simulink library "lpvlibrary"  (R2018b)
settings: Solver=ode45  StartTime=0.0  StopTime=10.0  RelTol=1e-3  EnableMultiTasking=on
values from neighbouring files (symbols this model uses):
  ns = order(pdG)    [lpvctrl.m]    (also in lpvctrl_2.m = size(akh,1); pcss_Sfunction.m = order(sys))
  nu = length(pdG.InputGroup.ctrl)    [lpvctrl.m]    (also in lpvctrl_2.m; test_lpvanalysis.m = 0:10)
  ny = 0    [lft_pass.m]    (also in lft_pgss.m; lft_ppss.m; lpvctrl.m = length(pdG.OutputGroup.meas); lpvctrl_2.m = length(pdG.OutputGroup.meas))
  pdG = pgss(Ap,Bp,C1,0,pv,fcn,'InputName','u','OutputName','y')    [TwoLink_nl.m]    (also in test_lpvanalysis.m = pgss(Acl,B,C,D,pv,func,     'InputName','u',     'OutputName)
undefined symbols (not defined in the file or in its folder): pass, pcss
libraries: $bdroot x10
Description:
  | LPV model library
settings Model: Creator=Fernando  LastModifiedBy=ferna
settings DataIOCC: LimitDataPoints=on
settings OptimizationCC: LifeSpan=inf
settings DebuggingCC: AllowSymbolicDim=off  SFUnexpectedBacktrackingDiag=warning  SFNoUnconditionalDefaultTransitionDiag=warning
settings SFSimCC: SimUseLocalCustomCode=off
settings RTWCC: RTWUseLocalCustomCode=off
settings CodeAppCC: StateflowObjectComments=on
settings GRTTargetCC: TargetLangStandard=C89/C90 (ANSI)  GeneratePreprocessorConditionals=Disable all
settings ConfigComp: CovMetricSettings=dw  CovHtmlReporting=on  CovSaveCumulativeToWorkspaceVar=on  CovSaveSingleToWorkspaceVar=on  CovExternalEMLEnable=off

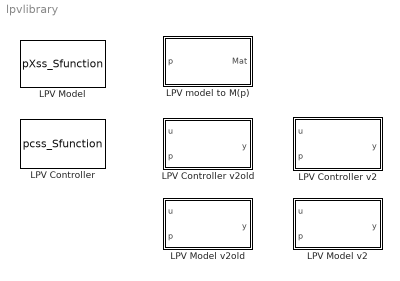
== system lpvlibrary ==
  LPV Controller : M-S-Function  FunctionName=pcss_Sfunction  Parameters=pdSys, x0  mask{pdSys=pcss('demo'), x0=0}
      mask prompts: pdSys "LPV controller (ctrlss)"; x0 "Initial Conditions"
      mask Display:
      | disp('')
      | port_label('input', 1, 'u')
      | port_label('input', 2, 'p')
      | port_label('output', 1, 'y')
  LPV Controller v2 : Subsystem  mask(LPV controller){pdK=pcss('demo'), x0=0}
      mask prompts: pdK "LPV Controller"; x0 "Initial conditions"
      mask help:
      | Online implementation of LPV controller for parameter dependent Lyapunov functions given in an object pcss.
      | Faster implementation than LPV controller block
      mask init:
      | % model dimensions
      | [ny,nu,ns] = size(pdK);
      | 
      | % Lyapunov function at par
      | flagX = isnumeric(pdK.xFcn);
      | flagY = isnumeric(pdK.yFcn);
      | 
      | % DirectFeedthrough flag
      | fDF = any(pdK.ctrller.D(:));
      | if fDF
      |     p1 = find_system(gcb);
      |     p2 = [p1{1} '/Du'];
      |     h1 = get_param(p2,'LineHandles');
      |     delete_line(h1.Outport);
      |     
      |     p1 = find_system(gcb);
      |     p2 = [p1{1} '/d0'];
      |     h1 = get_param(p2,'LineHandles');
      |     delete_line(h1.Outport)
      |     
      |     add_line(gcb,'Du/1','sb/2','autorouting','on');
      |     add_line(gcb,'d0/1','end/1','autorouting','on');
      |        
      | else
      |     p1 = find_system(gcb);
      |     p2 = [p1{1} '/Du'];
      |     h1 = get_param(p2,'LineHandles');
      |     delete_line(h1.Outport);
      |     
      |     p1 = find_system(gcb);
      |     p2 = [p1{1} '/d0'];
      |     h1 = get_param(p2,'LineHandles');
      |     delete_line(h1.Outport)
      |     
      |     add_line(gcb,'Du/1','end/1','autorouting','on');
      |     add_line(gcb,'d0/1','sb/2','autorouting','on');
      | end
      mask Display:
      | disp('pcss ctrller')
      | port_label('input', 1, 'u')
      | port_label('input', 2, 'p')
      | port_label('output', 1, 'y')
  LPV Controller v2old : Subsystem  mask(LPV controller){pdK=pcss('demo'), x0=0}
      mask prompts: pdK "LPV Controller"; x0 "Initial conditions"
      mask help:
      | Online implementation of LPV controller for parameter dependent Lyapunov functions given in an object pcss.
      | Faster implementation than LPV controller block
      mask init:
      | % model dimensions
      | [ny,nu,ns] = size(pdK);
      | 
      | % Lyapunov function at par
      | flagX = isnumeric(pdK.xFcn);
      | flagY = isnumeric(pdK.yFcn);
      | 
      | % DirectFeedthrough flag
      | fDF = any(pdK.D(:));
      | if fDF
      |     p1 = find_system(gcb);
      |     p2 = [p1{1} '/Du'];
      |     h1 = get_param(p2,'LineHandles');
      |     delete_line(h1.Outport);
      |     
      |     p1 = find_system(gcb);
      |     p2 = [p1{1} '/d0'];
      |     h1 = get_param(p2,'LineHandles');
      |     delete_line(h1.Outport)
      |     
      |     add_line(gcb,'Du/1','sb/2','autorouting','on');
      |     add_line(gcb,'d0/1','end/1','autorouting','on');
      |        
      | else
      |     p1 = find_system(gcb);
      |     p2 = [p1{1} '/Du'];
      |     h1 = get_param(p2,'LineHandles');
      |     delete_line(h1.Outport);
      |     
      |     p1 = find_system(gcb);
      |     p2 = [p1{1} '/d0'];
      |     h1 = get_param(p2,'LineHandles');
      |     delete_line(h1.Outport)
      |     
      |     add_line(gcb,'Du/1','end/1','autorouting','on');
      |     add_line(gcb,'d0/1','sb/2','autorouting','on');
      | end
      | 
      | set_param(gcb,'MaskHideContents','on')
      mask Display:
      | disp('pcss ctrller')
      | port_label('input', 1, 'u')
      | port_label('input', 2, 'p')
      | port_label('output', 1, 'y')
  LPV Model : M-S-Function  FunctionName=pXss_Sfunction  Parameters=pdSys, x0  mask{pdSys=pass(ss(ones(1,1,2)),[0 1]), x0=0}
      mask prompts: pdSys "LPV mode (pass, ppss)"; x0 "Initial conditions"
      mask Display:
      | disp('')
      | port_label('input', 1, 'u')
      | port_label('input', 2, 'p')
      | port_label('output', 1, 'y')
  LPV Model v2 : Subsystem  mask(LPV model){pdG=pdG, x0=0}
      mask prompts: pdG "LPV Model"; x0 "Initial conditions"
      mask help: Faster implementation of affine, general or polytopic LPV models given in an object pass, pgss or ppss
      mask init:
      | % model dimensions
      | [ny,nu,ns,np,nv] = size(pdG);
      | 
      | % interpolation 
      | type = class(pdG);
      | switch type
      |     case 'pass'
      |         fcn = [];
      |         
      |     case 'pgss'
      |         fcn = pdG.parfcn;
      |         
      |     case 'ppss'
      |         fcn = pdG.parset;
      | end
      | 
      | % model matrices
      | M = [pdG.A pdG.B;
      |      pdG.C pdG.D];
      | Mdata = reshape(M,(ns+ny)*(ns+nu),nv,1);
      | 
      | % DirectFeedthrough flag
      | fDF = any(pdG.D(:));
      | if fDF
      |     p1 = find_system(gcb);
      |     p2 = [p1{1} '/Du'];
      |     h1 = get_param(p2,'LineHandles');
      |     delete_line(h1.Outport);
      |     
      |     p1 = find_system(gcb);
      |     p2 = [p1{1} '/d0'];
      |     h1 = get_param(p2,'LineHandles');
      |     delete_line(h1.Outport)
      |     
      |     add_line(gcb,'Du/1','sb/2','autorouting','on');
      |     add_line(gcb,'d0/1','end/1','autorouting','on');
      |        
      | else
      |     p1 = find_system(gcb);
      |     p2 = [p1{1} '/Du'];
      |     h1 = get_param(p2,'LineHandles');
      |     delete_line(h1.Outport);
      |     
      |     p1 = find_system(gcb);
      |     p2 = [p1{1} '/d0'];
      |     h1 = get_param(p2,'LineHandles');
      |     delete_line(h1.Outport)
      |     
      |     add_line(gcb,'Du/1','end/1','autorouting','on');
      |     add_line(gcb,'d0/1','sb/2','autorouting','on');
      | end
      mask Display:
      | disp('LPV model')
      | port_label('input', 1, 'u')
      | port_label('input', 2, 'p')
      | port_label('output', 1, 'y')
  LPV Model v2old : Subsystem  mask(LPV model){pdG=pass(ss(ones(1,1,2)),[0 1]), x0=0}
      mask prompts: pdG "LPV Model"; x0 "Initial conditions"
      mask help: Faster implementation of affine, general or polytopic LPV models given in an object pass, pgss or ppss
      mask init:
      | % model dimensions
      | [ny,nu,ns,np,nv] = size(pdG);
      | 
      | % interpolation 
      | type = class(pdG);
      | switch type
      |     case 'pass'
      |         fcn = [];
      |         
      |     case 'pgss'
      |         fcn = pdG.parfcn;
      |         
      |     case 'ppss'
      |         fcn = pdG.parset;
      | end
      | 
      | % model matrices
      | M = [pdG.A pdG.B;
      |      pdG.C pdG.D];
      | Mdata = reshape(M,(ns+ny)*(ns+nu),nv,1);
      mask Display:
      | disp('LPV model')
      | port_label('input', 1, 'u')
      | port_label('input', 2, 'p')
      | port_label('output', 1, 'y')
  "LPV model to M(p) " : Subsystem  mask(LPV model to M(p)){pdG=pass(ss(ones(1,1,2)),[0 1])}
      mask prompts: pdG "LPV Model"
      mask help: Conversion of pass, ppss, pgss into a parameter dependent matrix
      mask init:
      | if isnumeric(pdG)
      |     % numeric matrix
      |     [ny,nu] = size(pdG);
      |     np = 1;
      |     nv = [ny ny];
      |     ns = 0;
      | 
      |     type = 'mat';
      |     fcn = 1;
      | 
      |     Mdata = pdG;
      |     
      | else
      |     % parameter dependent matrix
      |     [ny,nu,ns,np,nv] = size(pdG);
      |     
      |     type = class(pdG);
      |     switch type
      |         case 'pass'
      |             fcn = [];
      |             
      |         case 'pgss'
      |             fcn = pdG.parfcn;
      |             
      |         case 'ppss'
      |             fcn = pdG.parset;
      |     end
      |     
      |     M = [pdG.A pdG.B;
      |          pdG.C pdG.D];
      |     Mdata = reshape(M,(ns+ny)*(ns+nu),nv,1);
      |     
      | end
      mask Display:
      | disp('M(p)')
      | port_label('input', 1, 'p')
      | port_label('output', 1, 'Mat')

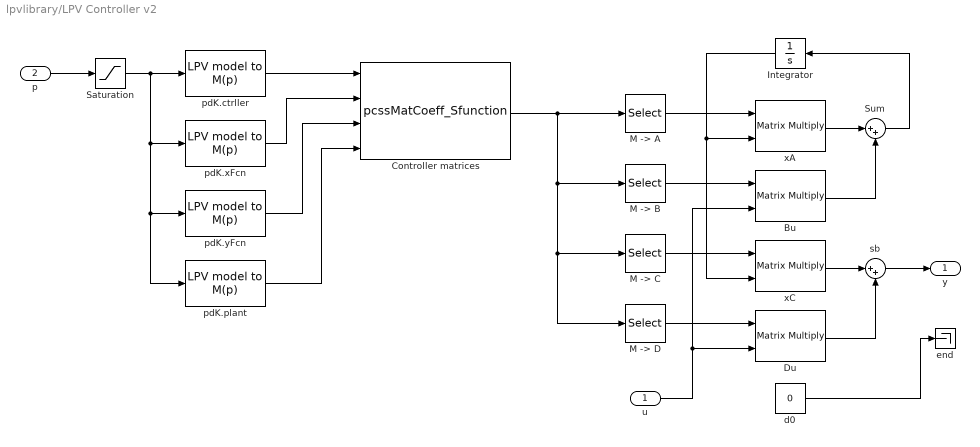
== system lpvlibrary/LPV Controller v2 ==
  "u " : Inport
  p : Inport  Port=2
  Bu : Product  Inputs=**  Multiplication=Matrix(*)
  Controller matrices : M-S-Function  FunctionName=pcssMatCoeff_Sfunction  Parameters=ns, ny, nu, flagX, flagY
  Du : Product  Inputs=**  Multiplication=Matrix(*)
  Integrator : Integrator  InitialCondition=x0
  "M -> A" : Selector  NumberOfDimensions=2  InputPortWidth=3  IndexOptions=Index vector (dialog),Index vector (dialog)  Indices=1:ns,1:ns  OutputSizes=1,1
  "M -> B" : Selector  NumberOfDimensions=2  InputPortWidth=3  IndexOptions=Index vector (dialog),Index vector (dialog)  Indices=1:ns,1+ns:ns+nu  OutputSizes=1,1
  "M -> C" : Selector  NumberOfDimensions=2  InputPortWidth=3  IndexOptions=Index vector (dialog),Index vector (dialog)  Indices=1+ns:ns+ny,1:ns  OutputSizes=1,1
  "M -> D" : Selector  NumberOfDimensions=2  InputPortWidth=3  IndexOptions=Index vector (dialog),Index vector (dialog)  Indices=1+ns:ns+ny,1+ns:ns+nu  OutputSizes=1,1
  Saturation : Saturate  UpperLimit=pdK.parset.range(:,2)  LowerLimit=pdK.parset.range(:,1)
  Sum : Sum  Inputs=|++
  d0 : Constant  Value=0
  end : Terminator
  pdK.ctrller : $bdroot/LPV model to M(p)   pdG=pdK.ctrller
  pdK.plant : $bdroot/LPV model to M(p)   pdG=pdK.plant
  "pdK.xFcn " : $bdroot/LPV model to M(p)   pdG=pdK.xFcn
  pdK.yFcn : $bdroot/LPV model to M(p)   pdG=pdK.yFcn
  sb : Sum  Inputs=|++
  xA : Product  Inputs=**  Multiplication=Matrix(*)
  xC : Product  Inputs=**  Multiplication=Matrix(*)
  y : Outport
  wires:
  Saturation/1 -> "pdK.xFcn "/1, pdK.yFcn/1, pdK.plant/1, pdK.ctrller/1
  pdK.plant/1 -> Controller matrices/4
  pdK.yFcn/1 -> Controller matrices/3
  "pdK.xFcn "/1 -> Controller matrices/2
  pdK.ctrller/1 -> Controller matrices/1
  p/1 -> Saturation/1
  Integrator/1 -> xC/2, xA/2
  Bu/1 -> Sum/2
  "u "/1 -> Bu/2, Du/2
  Sum/1 -> Integrator/1
  Controller matrices/1 -> "M -> D"/1, "M -> C"/1, "M -> B"/1, "M -> A"/1
  "M -> B"/1 -> Bu/1
  "M -> A"/1 -> xA/1
  sb/1 -> y/1
  "M -> D"/1 -> Du/1
  "M -> C"/1 -> xC/1
  xC/1 -> sb/1
  xA/1 -> Sum/1
  Du/1 -> sb/2
  d0/1 -> end/1

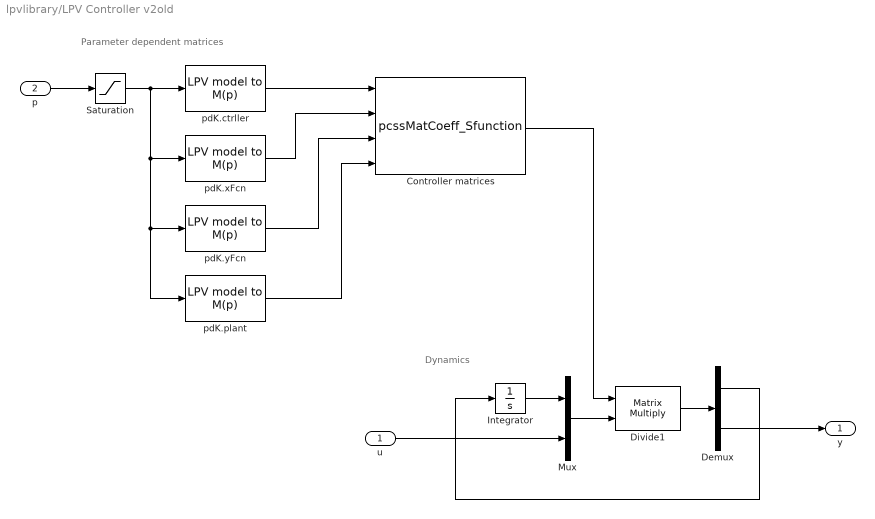
== system lpvlibrary/LPV Controller v2old ==
  note: Dynamics
  note: Parameter dependent matrices
  "u " : Inport  PortDimensions=nu
  p : Inport  Port=2
  Controller matrices : M-S-Function  FunctionName=pcssMatCoeff_Sfunction  Parameters=ns, ny, nu, flagX, flagY
  Demux : Demux  Outputs=[ns, ny]
  Divide1 : Product  Inputs=**  Multiplication=Matrix(*)
  Integrator : Integrator
  Mux : Mux  Inputs=[ns, nu]
  Saturation : Saturate  UpperLimit=pdK.parset.range(:,2)  LowerLimit=pdK.parset.range(:,1)
  pdK.ctrller : $bdroot/LPV model to M(p)   pdG=pdK.ctrller
  pdK.plant : $bdroot/LPV model to M(p)   pdG=pdK.plant
  "pdK.xFcn " : $bdroot/LPV model to M(p)   pdG=pdK.xFcn
  pdK.yFcn : $bdroot/LPV model to M(p)   pdG=pdK.yFcn
  y : Outport
  wires:
  "u "/1 -> Mux/2
  Integrator/1 -> Mux/1
  Demux/1 -> Integrator/1
  Demux/2 -> y/1
  Divide1/1 -> Demux/1
  Mux/1 -> Divide1/2
  Controller matrices/1 -> Divide1/1
  p/1 -> Saturation/1
  pdK.ctrller/1 -> Controller matrices/1
  "pdK.xFcn "/1 -> Controller matrices/2
  pdK.yFcn/1 -> Controller matrices/3
  pdK.plant/1 -> Controller matrices/4
  Saturation/1 -> pdK.ctrller/1, pdK.plant/1, pdK.yFcn/1, "pdK.xFcn "/1

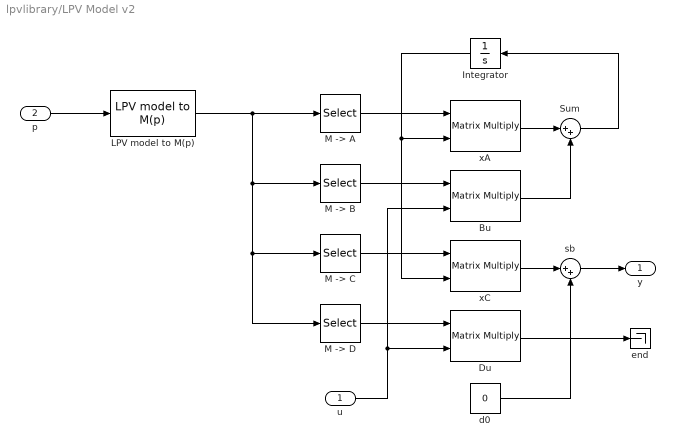
== system lpvlibrary/LPV Model v2 ==
  "u " : Inport
  p : Inport  Port=2
  Bu : Product  Inputs=**  Multiplication=Matrix(*)
  Du : Product  Inputs=**  Multiplication=Matrix(*)
  Integrator : Integrator  InitialCondition=x0
  LPV model to M(p) : $bdroot/LPV model to M(p)   pdG=pdG
  "M -> A" : Selector  NumberOfDimensions=2  InputPortWidth=3  IndexOptions=Index vector (dialog),Index vector (dialog)  Indices=1:ns,1:ns  OutputSizes=1,1
  "M -> B" : Selector  NumberOfDimensions=2  InputPortWidth=3  IndexOptions=Index vector (dialog),Index vector (dialog)  Indices=1:ns,1+ns:ns+nu  OutputSizes=1,1
  "M -> C" : Selector  NumberOfDimensions=2  InputPortWidth=3  IndexOptions=Index vector (dialog),Index vector (dialog)  Indices=1+ns:ns+ny,1:ns  OutputSizes=1,1
  "M -> D" : Selector  NumberOfDimensions=2  InputPortWidth=3  IndexOptions=Index vector (dialog),Index vector (dialog)  Indices=1+ns:ns+ny,1+ns:ns+nu  OutputSizes=1,1
  Sum : Sum  Inputs=|++
  d0 : Constant  Value=0
  end : Terminator
  sb : Sum  Inputs=|++
  xA : Product  Inputs=**  Multiplication=Matrix(*)
  xC : Product  Inputs=**  Multiplication=Matrix(*)
  y : Outport
  wires:
  p/1 -> LPV model to M(p)/1
  LPV model to M(p)/1 -> "M -> D"/1, "M -> C"/1, "M -> B"/1, "M -> A"/1
  "M -> A"/1 -> xA/1
  Integrator/1 -> xC/2, xA/2
  "M -> B"/1 -> Bu/1
  "u "/1 -> Bu/2, Du/2
  xA/1 -> Sum/1
  Bu/1 -> Sum/2
  Sum/1 -> Integrator/1
  "M -> C"/1 -> xC/1
  xC/1 -> sb/1
  sb/1 -> y/1
  "M -> D"/1 -> Du/1
  Du/1 -> end/1
  d0/1 -> sb/2

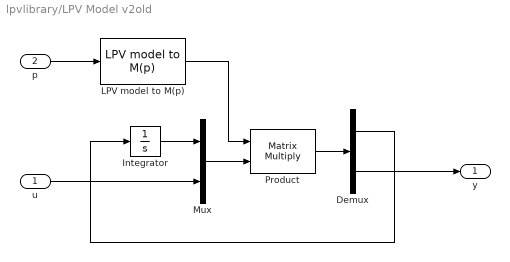
== system lpvlibrary/LPV Model v2old ==
  "u " : Inport
  p : Inport  Port=2
  Demux : Demux  Outputs=[ns, ny]
  Integrator : Integrator  InitialCondition=x0
  "LPV model to M(p) " : $bdroot/LPV model to M(p)   pdG=pdG
  Mux : Mux  Inputs=[ns, nu]
  Product : Product  Inputs=**  Multiplication=Matrix(*)
  y : Outport
  wires:
  "u "/1 -> Mux/2
  Integrator/1 -> Mux/1
  Demux/1 -> Integrator/1
  Demux/2 -> y/1
  Product/1 -> Demux/1
  Mux/1 -> Product/2
  p/1 -> "LPV model to M(p) "/1
  "LPV model to M(p) "/1 -> Product/1

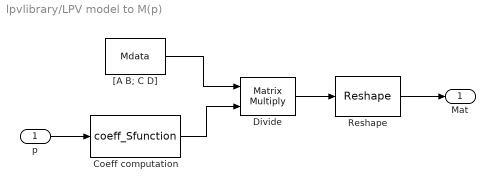
== system lpvlibrary/LPV model to M(p)  ==
  p : Inport
  Coeff computation : M-S-Function  FunctionName=coeff_Sfunction  Parameters=np, nv, fcn, type
  Divide : Product  Inputs=**  Multiplication=Matrix(*)
  Reshape : Reshape  OutputDimensionality=Customize  OutputDimensions=[ns+ny, ns+nu, 1]
  "[A B; C D]" : Constant  Value=Mdata  VectorParams1D=off
  Mat : Outport
  wires:
  Divide/1 -> Reshape/1
  p/1 -> Coeff computation/1
  Coeff computation/1 -> Divide/2
  "[A B; C D]"/1 -> Divide/1
  Reshape/1 -> Mat/1
